simulink model "PID_cascaded"  (R2017b)
settings: Solver=ode4  StartTime=0.0  StopTime=0.40905  FixedStep=0.001  RelTol=1e-3
settings Model: Creator=84935  LastModifiedBy=84935

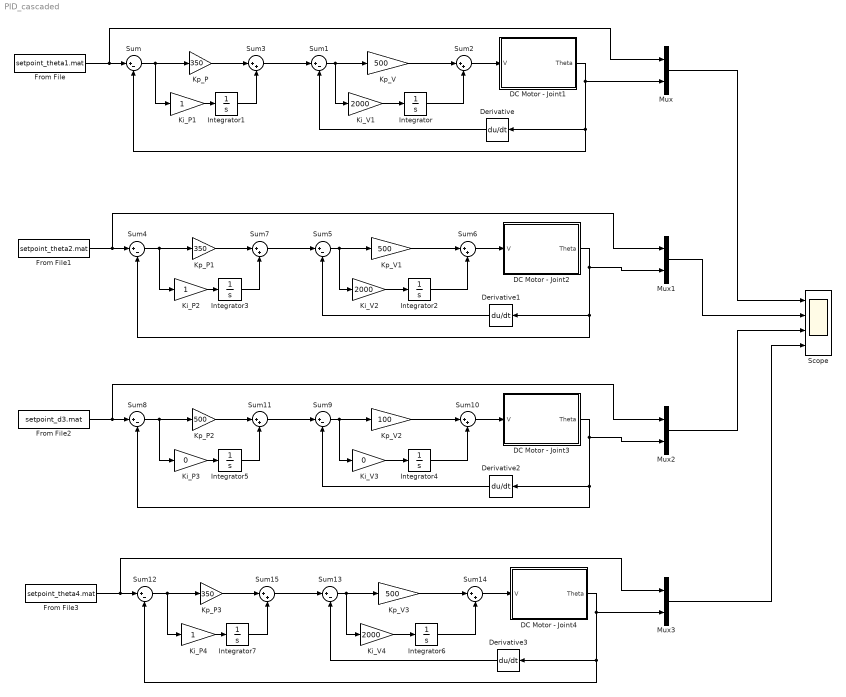
== system PID_cascaded ==
  DC Motor - Joint1 : Subsystem  mask{L=0.012342, R=3.2645, Ki=1.1895, Jeff=0.01829, Beff=0.019, Kb=1.1895, N=200}
  DC Motor - Joint2 : Subsystem  mask{L=0.012342, R=3.2645, Ki=1.1895, Jeff=0.01829, Beff=0.019, Kb=1.1895, N=100}
  DC Motor - Joint3 : Subsystem  mask{L=0.012342, R=3.2645, Ki=1.1895, Jeff=0.01829, Beff=0.019, Kb=1.1895, N=100}
  DC Motor - Joint4 : Subsystem  mask{L=0.012342, R=3.2645, Ki=1.1895, Jeff=0.01829, Beff=0.019, Kb=1.1895, N=50}
  Derivative{,1..3} (4 alike) : Derivative
  From File : FromFile  FileName=setpoint_theta1.mat  SampleTime=0
  From File1 : FromFile  FileName=setpoint_theta2.mat  SampleTime=0
  From File2 : FromFile  FileName=setpoint_d3.mat  SampleTime=0
  From File3 : FromFile  FileName=setpoint_theta4.mat  SampleTime=0
  Integrator{,1..7} (8 alike) : Integrator
  Ki_P1 : Gain
  Ki_P2 : Gain
  Ki_P3 : Gain  Gain=0
  Ki_P4 : Gain
  Ki_V1 : Gain  Gain=2000
  Ki_V2 : Gain  Gain=2000
  Ki_V3 : Gain  Gain=0
  Ki_V4 : Gain  Gain=2000
  Kp_P : Gain  Gain=350
  Kp_P1 : Gain  Gain=350
  Kp_P2 : Gain  Gain=500
  Kp_P3 : Gain  Gain=350
  Kp_V : Gain  Gain=500
  Kp_V1 : Gain  Gain=500
  Kp_V2 : Gain  Gain=100
  Kp_V3 : Gain  Gain=500
  Mux{,1..3} (4 alike) : Mux  Inputs=2
  Scope : Scope  NumInputPorts=4
  Sum{,1,4..5,8..9,12..13} (8 alike) : Sum  Inputs=|+-
  Sum{2..3,6..7,10..11,14..15} (8 alike) : Sum  Inputs=|++
  wires:
  Derivative/1 -> Sum1/2
  Sum1/1 -> Kp_V/1, Ki_V1/1
  Kp_V/1 -> Sum2/1
  Integrator/1 -> Sum2/2
  Sum3/1 -> Sum1/1
  Sum2/1 -> DC Motor - Joint1/1(V)
  Ki_V1/1 -> Integrator/1
  Sum/1 -> Ki_P1/1, Kp_P/1
  Integrator1/1 -> Sum3/2
  Kp_P/1 -> Sum3/1
  DC Motor - Joint1/1(Theta) -> Mux/2, Sum/2, Derivative/1
  From File/1 -> Mux/1, Sum/1
  Ki_P1/1 -> Integrator1/1
  Kp_P1/1 -> Sum7/1
  Sum4/1 -> Ki_P2/1, Kp_P1/1
  Integrator3/1 -> Sum7/2
  Ki_P2/1 -> Integrator3/1
  From File1/1 -> Mux1/1, Sum4/1
  Integrator2/1 -> Sum6/2
  Kp_V1/1 -> Sum6/1
  Derivative1/1 -> Sum5/2
  Ki_V2/1 -> Integrator2/1
  Sum5/1 -> Kp_V1/1, Ki_V2/1
  DC Motor - Joint2/1(Theta) -> Mux1/2, Sum4/2, Derivative1/1
  Sum7/1 -> Sum5/1
  Sum6/1 -> DC Motor - Joint2/1(V)
  Kp_P2/1 -> Sum11/1
  Sum8/1 -> Ki_P3/1, Kp_P2/1
  Integrator5/1 -> Sum11/2
  Ki_P3/1 -> Integrator5/1
  From File2/1 -> Mux2/1, Sum8/1
  Integrator4/1 -> Sum10/2
  Kp_V2/1 -> Sum10/1
  Derivative2/1 -> Sum9/2
  Ki_V3/1 -> Integrator4/1
  Sum9/1 -> Kp_V2/1, Ki_V3/1
  DC Motor - Joint3/1(Theta) -> Mux2/2, Sum8/2, Derivative2/1
  Sum11/1 -> Sum9/1
  Sum10/1 -> DC Motor - Joint3/1(V)
  Kp_P3/1 -> Sum15/1
  Sum12/1 -> Ki_P4/1, Kp_P3/1
  Integrator7/1 -> Sum15/2
  Ki_P4/1 -> Integrator7/1
  From File3/1 -> Mux3/1, Sum12/1
  Integrator6/1 -> Sum14/2
  Kp_V3/1 -> Sum14/1
  Derivative3/1 -> Sum13/2
  Ki_V4/1 -> Integrator6/1
  Sum13/1 -> Kp_V3/1, Ki_V4/1
  DC Motor - Joint4/1(Theta) -> Mux3/2, Sum12/2, Derivative3/1
  Sum15/1 -> Sum13/1
  Sum14/1 -> DC Motor - Joint4/1(V)
  Mux/1 -> Scope/1
  Mux1/1 -> Scope/2
  Mux2/1 -> Scope/3
  Mux3/1 -> Scope/4

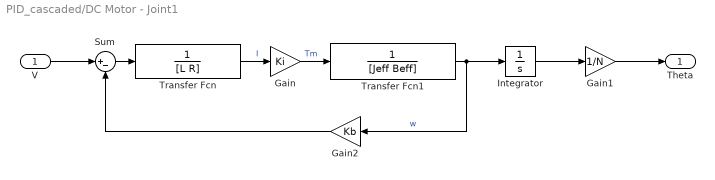
== system PID_cascaded/DC Motor - Joint1 ==
  V : Inport
  Gain : Gain  Gain=Ki
  Gain1 : Gain  Gain=1/N
  Gain2 : Gain  Gain=Kb
  Integrator : Integrator
  Sum : Sum  Inputs=|+-
  Transfer Fcn : TransferFcn  Denominator=[L R]
  Transfer Fcn1 : TransferFcn  Denominator=[Jeff Beff]
  Theta : Outport
  wires:
  Integrator/1 -> Gain1/1
  Transfer Fcn1/1 -> Integrator/1, Gain2/1  "w"
  V/1 -> Sum/1
  Gain2/1 -> Sum/2
  Gain/1 -> Transfer Fcn1/1  "Tm"
  Gain1/1 -> Theta/1
  Sum/1 -> Transfer Fcn/1
  Transfer Fcn/1 -> Gain/1  "I"

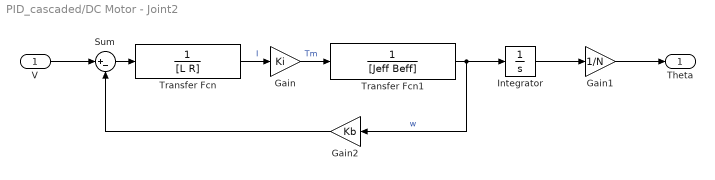
== system PID_cascaded/DC Motor - Joint2 ==
  V : Inport
  Gain : Gain  Gain=Ki
  Gain1 : Gain  Gain=1/N
  Gain2 : Gain  Gain=Kb
  Integrator : Integrator
  Sum : Sum  Inputs=|+-
  Transfer Fcn : TransferFcn  Denominator=[L R]
  Transfer Fcn1 : TransferFcn  Denominator=[Jeff Beff]
  Theta : Outport
  wires:
  Integrator/1 -> Gain1/1
  Transfer Fcn1/1 -> Integrator/1, Gain2/1  "w"
  V/1 -> Sum/1
  Gain2/1 -> Sum/2
  Gain/1 -> Transfer Fcn1/1  "Tm"
  Gain1/1 -> Theta/1
  Sum/1 -> Transfer Fcn/1
  Transfer Fcn/1 -> Gain/1  "I"

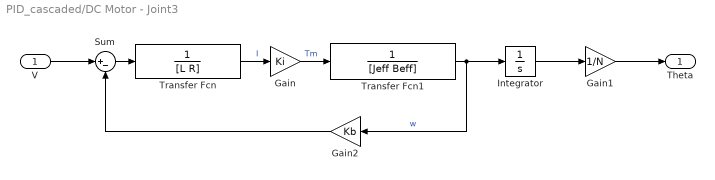
== system PID_cascaded/DC Motor - Joint3 ==
  V : Inport
  Gain : Gain  Gain=Ki
  Gain1 : Gain  Gain=1/N
  Gain2 : Gain  Gain=Kb
  Integrator : Integrator
  Sum : Sum  Inputs=|+-
  Transfer Fcn : TransferFcn  Denominator=[L R]
  Transfer Fcn1 : TransferFcn  Denominator=[Jeff Beff]
  Theta : Outport
  wires:
  Integrator/1 -> Gain1/1
  Transfer Fcn1/1 -> Integrator/1, Gain2/1  "w"
  V/1 -> Sum/1
  Gain2/1 -> Sum/2
  Gain/1 -> Transfer Fcn1/1  "Tm"
  Gain1/1 -> Theta/1
  Sum/1 -> Transfer Fcn/1
  Transfer Fcn/1 -> Gain/1  "I"

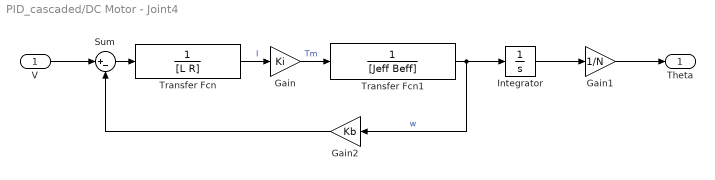
== system PID_cascaded/DC Motor - Joint4 ==
  V : Inport
  Gain : Gain  Gain=Ki
  Gain1 : Gain  Gain=1/N
  Gain2 : Gain  Gain=Kb
  Integrator : Integrator
  Sum : Sum  Inputs=|+-
  Transfer Fcn : TransferFcn  Denominator=[L R]
  Transfer Fcn1 : TransferFcn  Denominator=[Jeff Beff]
  Theta : Outport
  wires:
  Integrator/1 -> Gain1/1
  Transfer Fcn1/1 -> Integrator/1, Gain2/1  "w"
  V/1 -> Sum/1
  Gain2/1 -> Sum/2
  Gain/1 -> Transfer Fcn1/1  "Tm"
  Gain1/1 -> Theta/1
  Sum/1 -> Transfer Fcn/1
  Transfer Fcn/1 -> Gain/1  "I"
